simulink model "testmodel1"  (R2019b)
settings: Solver=ode3  StartTime=0.0  StopTime=10.0  RelTol=1e-3  EnableMultiTasking=on
settings Model: Creator=Bryan  LastModifiedBy=bhisma
settings DataIOCC: LimitDataPoints=on  SaveFormat=Array  ReturnWorkspaceOutputs=off
settings OptimizationCC: LifeSpan=inf
settings DebuggingCC: SolverPrmCheckMsg=warning  SFUnexpectedBacktrackingDiag=warning  SFNoUnconditionalDefaultTransitionDiag=warning  SFExecutionAtInitializationDiag=none  ArithmeticOperatorsInVariantConditions=warning
settings HardwareCC: ProdBitPerPointer=32  ProdBitPerSizeT=32  ProdBitPerPtrDiffT=32  ProdLargestAtomicFloat=None  ProdIntDivRoundTo=Undefined  ProdEndianess=Unspecified  ProdWordSize=32  ProdHWDeviceType=32-bit Generic
settings ModelReferenceCC: PropagateSignalLabelsOutOfModel=off
settings SFSimCC: SimUseLocalCustomCode=off  CustomCodeUndefinedFunction=UseInterfaceOnly
settings RTWCC: Description=Create Visual C/C++ Solution File for Simulink Coder  TemplateMakefile=RTW.MSVCBuild  GenerateReport=on  RTWUseLocalCustomCode=off  LaunchReport=on
settings CodeAppCC: ForceParamTrailComments=on  StateflowObjectComments=on  MATLABSourceComments=on
settings GRTTargetCC: TargetLangStandard=C89/C90 (ANSI)  GeneratePreprocessorConditionals=Disable all  MatFileLogging=off
settings ConfigComp: CovMetricSettings=dw  CovHtmlReporting=on  CovSaveCumulativeToWorkspaceVar=on  CovSaveSingleToWorkspaceVar=on  CovExternalEMLEnable=off  CovSFcnEnable=off

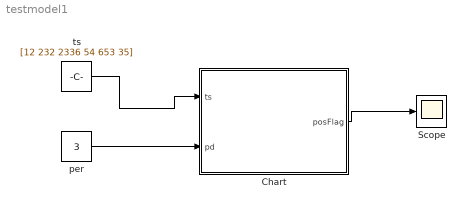
== system testmodel1 ==
  Chart : Stateflow chart  TreatAsAtomicUnit=on
  Scope : Scope
  "per " : Constant  Value=3
  ts : Constant  Value=[12 232 2336 54 653 35]  VectorParams1D=off
  wires:
  Chart/1(posFlag) -> Scope/1
  ts/1 -> Chart/1(ts)
  "per "/1 -> Chart/2(pd)

== stateflow chart testmodel1/Chart ==
  state buy
    en: posFlag=1
  state sell
    en: posFlag=-1
  (default) -> (junction 7) : {avg=testMovAvg(ts,pd)}
  sell -> (junction 7)
  (junction 7) -> sell [order 2] : [avg>50]
  buy -> (junction 7)
  (junction 7) -> buy [order 1] : [avg<50]
  data: x function_input; ped function_input =ped; avgNum function_output; posFlag output size=1; ts input; pd input; avg local
  function avgNum=testMovAvg(x,ped):
    | function avgNum=testMovAvg(x,ped)
    | %ensure out variable does not cofnflict with other model objects 
    | %this directive is need to add input and output on Stateflow chart block!
    | %#codegen
    | avgNum = 0; %must define for code generation
    | avgNum = sum(x)/ped;
